simulink model "SystemeCompletProcedural"  (R2019b)
settings: Solver=FixedStepAuto  StartTime=0.0  StopTime=7  FixedStep=0.0001  RelTol=1e-3
libraries: dspsrcs4 x2
settings Model: Creator=jeanz  LastModifiedBy=maxim

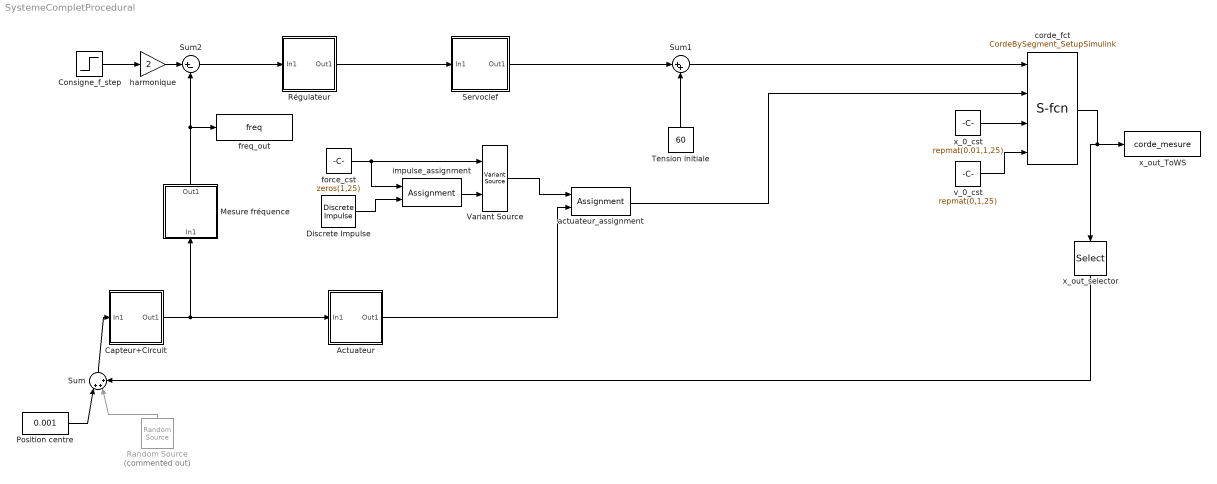
== system SystemeCompletProcedural ==
  Actuateur : Subsystem
  Capteur+Circuit : Subsystem
  Consigne_f_step : Step  Time=3  Before=100  After=110  SampleTime=0
  Discrete Impulse : dspsrcs4/Discrete  Impulse  Delay=0  SampleTime=0.1  FrameSample=1  OutputFrames=off  dataType=double  isSigned=on  wordLen=16  udDataType=sfix(16)  fracBitsMode=Best precision  numFracBits=15  OutDataTypeStr=double  LastOutDataTypeStr=double
  Mesure fréquence : Subsystem
  Position centre : Constant  Value=0.001
  Random Source : dspsrcs4/Random Source  Commented=on  SrcType=Uniform  NormMethod=Ziggurat  CltLength=12  MinVal=-0.0001  MaxVal=0.0001  MeanVal=0  VarVal=1  RepMode=Not repeatable  rawSeed=1  IsInherit=off  SampMode=Discrete  SampTime=1  SampFrame=1  DataType=Double  OutComplex=Real  OutputFrames=off
  Régulateur : Subsystem
  Servoclef : Subsystem
  Sum : Sum  Inputs=|+++
  Sum1 : Sum  Inputs=|++
  Sum2 : Sum  Inputs=|+-
  Tension initiale : Constant  Value=60
  Variant Source : VariantSource  VariantControlMode=Label  LabelModeActiveChoice=ImpulseOff
  actuateur_assignment : Assignment  DiagnosticForDimensions=Warning  IndexOptions=Starting index (dialog)  Indices=7  OutputSizes=1
  corde_fct : M-S-Function  FunctionName=CordeBySegment_SetupSimulink  Parameters=3.251620e-03, 4.430000e-01, 3.260000e-02, 25, 1.000000e-04
  force_cst : Constant  Value=zeros(1,25)
  freq_out : ToWorkspace  VariableName=freq  SaveFormat=Timeseries  SampleTime=-1
  harmonique : Gain  Gain=2
  impulse_assignment : Assignment  DiagnosticForDimensions=Warning  IndexOptions=Starting index (dialog)  Indices=13  OutputSizes=1
  v_0_cst : Constant  Value=repmat(0,1,25)
  x_0_cst : Constant  Value=repmat(0.01,1,25)
  x_out_ToWS : ToWorkspace  VariableName=corde_mesure  SaveFormat=Timeseries  SampleTime=-1
  x_out_selector : Selector  IndexOptions=Starting index (dialog)  Indices=20  OutputSizes=1
  wires:
  actuateur_assignment/1 -> corde_fct/2
  corde_fct/1 -> x_out_ToWS/1, x_out_selector/1
  Capteur+Circuit/1(Out1) -> Mesure fréquence/1(In1), Actuateur/1(In1)
  Mesure fréquence/1(Out1) -> Sum2/2, freq_out/1
  Sum/1 -> Capteur+Circuit/1(In1)
  Position centre/1 -> Sum/1
  Tension initiale/1 -> Sum1/2
  Servoclef/1(Out1) -> Sum1/1
  Random Source/1 -> Sum/2
  Consigne_f_step/1 -> harmonique/1
  Régulateur/1(Out1) -> Servoclef/1(In1)
  Sum2/1 -> Régulateur/1(In1)
  x_out_selector/1 -> Sum/3
  Sum1/1 -> corde_fct/1
  x_0_cst/1 -> corde_fct/3
  v_0_cst/1 -> corde_fct/4
  impulse_assignment/1 -> Variant Source/2
  Actuateur/1(Out1) -> actuateur_assignment/2
  force_cst/1 -> impulse_assignment/1, Variant Source/1
  Discrete Impulse/1 -> impulse_assignment/2
  Variant Source/1 -> actuateur_assignment/1
  harmonique/1 -> Sum2/1

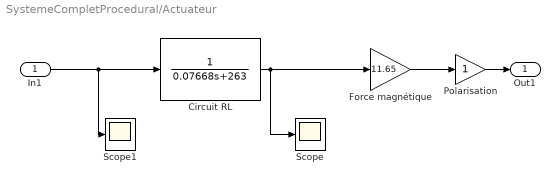
== system SystemeCompletProcedural/Actuateur ==
  In1 : Inport
  Circuit RL : TransferFcn  Denominator=[0.07668 263]
  Force magnétique : Gain  Gain=11.65
  Polarisation : Gain
  Scope : Scope
  Scope1 : Scope
  Out1 : Outport
  wires:
  Force magnétique/1 -> Polarisation/1
  Circuit RL/1 -> Force magnétique/1, Scope/1
  In1/1 -> Scope1/1, Circuit RL/1
  Polarisation/1 -> Out1/1

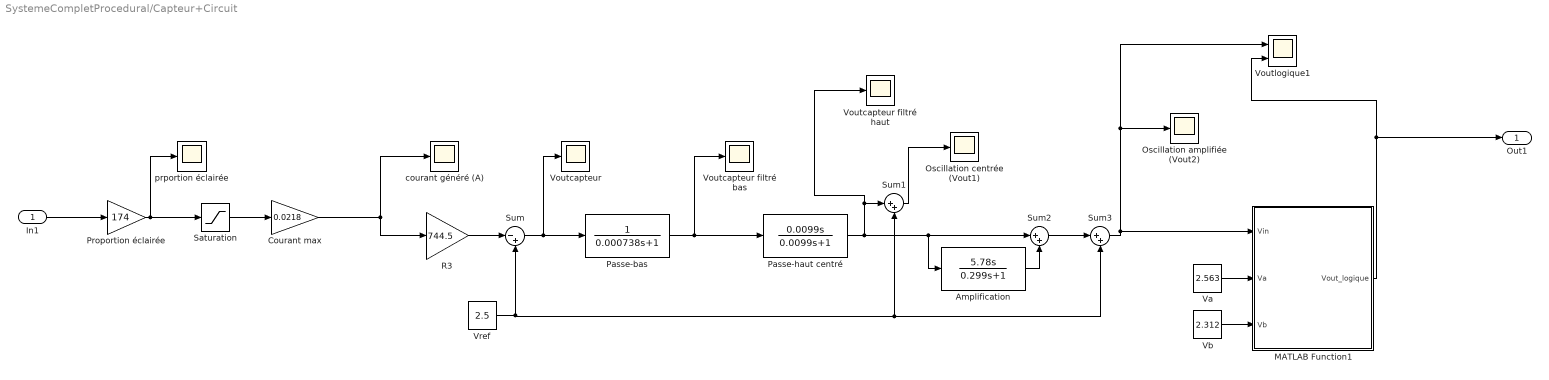
== system SystemeCompletProcedural/Capteur+Circuit ==
  In1 : Inport
  "Amplification " : TransferFcn  Numerator=[5.78 0]  Denominator=[0.299 1]
  Courant max : Gain  Gain=0.0218
  MATLAB Function1 : MATLAB Function  TreatAsAtomicUnit=on
  "Oscillation amplifiée (Vout2) " : Scope
  Oscillation centrée (Vout1) : Scope
  Passe-bas : TransferFcn  Denominator=[0.000738 1]
  "Passe-haut centré " : TransferFcn  Numerator=[0.0099 0]  Denominator=[0.0099 1]
  Proportion éclairée : Gain  Gain=174
  R3 : Gain  Gain=744.5
  Saturation : Saturate  UpperLimit=0.497  LowerLimit=0
  Sum : Sum  Inputs=|-+
  Sum1 : Sum  Inputs=|++
  Sum2 : Sum  Inputs=|++
  Sum3 : Sum  Inputs=|++
  "Va " : Constant  Value=2.563
  Vb : Constant  Value=2.312
  "Voutcapteur " : Scope
  Voutcapteur filtré bas : Scope
  Voutcapteur filtré haut : Scope
  Voutlogique1 : Scope  NumInputPorts=2
  "Vref " : Constant  Value=2.5
  "courant généré (A) " : Scope
  prportion éclairée : Scope
  Out1 : Outport
  wires:
  "Amplification "/1 -> Sum2/2
  Sum3/1 -> Voutlogique1/1, "Oscillation amplifiée (Vout2) "/1, MATLAB Function1/1(Vin)
  "Vref "/1 -> Sum/2, Sum3/2, Sum1/2
  Sum/1 -> "Voutcapteur "/1, Passe-bas/1
  R3/1 -> Sum/1
  "Passe-haut centré "/1 -> Sum2/1, "Amplification "/1, Voutcapteur filtré haut/1, Sum1/1
  Vb/1 -> MATLAB Function1/3(Vb)
  Passe-bas/1 -> Voutcapteur filtré bas/1, "Passe-haut centré "/1
  Sum2/1 -> Sum3/1
  Sum1/1 -> Oscillation centrée (Vout1)/1
  MATLAB Function1/1(Vout_logique) -> Out1/1, Voutlogique1/2
  "Va "/1 -> MATLAB Function1/2(Va)
  Saturation/1 -> Courant max/1
  Proportion éclairée/1 -> Saturation/1, prportion éclairée/1
  Courant max/1 -> R3/1, "courant généré (A) "/1
  In1/1 -> Proportion éclairée/1

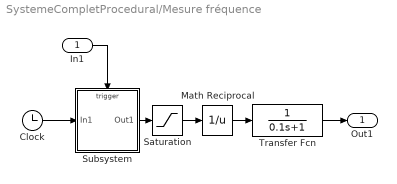
== system SystemeCompletProcedural/Mesure fréquence ==
  In1 : Inport
  Clock : Clock
  Math Reciprocal : Math  Operator=reciprocal  SaturateOnIntegerOverflow=on
  Saturation : Saturate  UpperLimit=1  LowerLimit=0.001
  Subsystem : Subsystem
  Transfer Fcn : TransferFcn  Denominator=[0.1 1]
  Out1 : Outport
  wires:
  In1/1 -> Subsystem/Trigger
  Clock/1 -> Subsystem/1(In1)
  Subsystem/1(Out1) -> Saturation/1
  Saturation/1 -> Math Reciprocal/1
  Math Reciprocal/1 -> Transfer Fcn/1
  Transfer Fcn/1 -> Out1/1

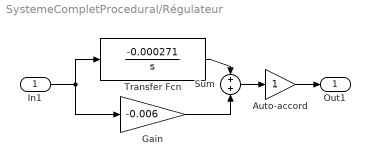
== system SystemeCompletProcedural/Régulateur ==
  In1 : Inport
  Auto-accord : Gain
  Gain : Gain  Gain=-0.006
  Sum : Sum  Inputs=+|+
  Transfer Fcn : TransferFcn  Numerator=[-0.000271]  Denominator=[1 0]
  Out1 : Outport
  wires:
  In1/1 -> Gain/1, Transfer Fcn/1
  Sum/1 -> Auto-accord/1
  Transfer Fcn/1 -> Sum/1
  Gain/1 -> Sum/2
  Auto-accord/1 -> Out1/1

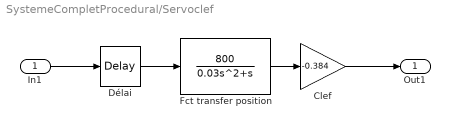
== system SystemeCompletProcedural/Servoclef ==
  In1 : Inport
  Clef : Gain  Gain=-0.384
  Délai : TransportDelay  DelayTime=0.01
  Fct transfer position : TransferFcn  Numerator=[800]  Denominator=[0.03 1 0]
  Out1 : Outport
  wires:
  Fct transfer position/1 -> Clef/1
  Clef/1 -> Out1/1
  Délai/1 -> Fct transfer position/1
  In1/1 -> Délai/1

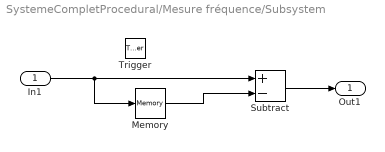
== system SystemeCompletProcedural/Mesure fréquence/Subsystem ==
  In1 : Inport
  Trigger : TriggerPort  VariantControl=Variant  PortDimensions=1
  Memory : Memory  InheritSampleTime=on
  Subtract : Sum  Inputs=+-
  Out1 : Outport
  wires:
  In1/1 -> Memory/1, Subtract/1
  Memory/1 -> Subtract/2
  Subtract/1 -> Out1/1

== matlab function SystemeCompletProcedural/Capteur+Circuit/MATLAB Function1 ==
  data: Vin input; Vout_logique output; Va input; Vb input
function Vout_logique = fcn(Vin, Va, Vb)

Vout_logique = 0;
if Vin > Va && Vout_logique == 5
    Vout_logique = 0;
end
if Vin < Vb && Vout_logique == 0
    Vout_logique = 5;
end
end
